simulink model "simulation_three_motors"  (R2022a)
settings: Solver=FixedStepAuto  StartTime=0.0  StopTime=inf  FixedStep=Ts  RelTol=1e-3
libraries: slDxl_lib_old x8
settings Model: Creator=jeihunl  LastModifiedBy=Matija
settings SolverCC: AlgebraicLoopSolver=TrustRegion
settings DataIOCC: ReturnWorkspaceOutputs=off
settings OptimizationCC: LifeSpan=inf
settings DebuggingCC: UnconnectedInputMsg=warning  UnconnectedOutputMsg=warning  UnconnectedLineMsg=warning  SFExecutionAtInitializationDiag=none  SFMachineParentedDataDiag=warning  ArithmeticOperatorsInVariantConditions=warning
settings HardwareCC: ProdBitPerSizeT=32  ProdBitPerPtrDiffT=32  ProdWordSize=32  ProdHWDeviceType=Specified
settings SFSimCC: SimUseLocalCustomCode=off  CustomCodeUndefinedFunction=UseInterfaceOnly
settings RTWCC: RTWUseLocalCustomCode=off
settings CodeAppCC: StateflowObjectComments=on

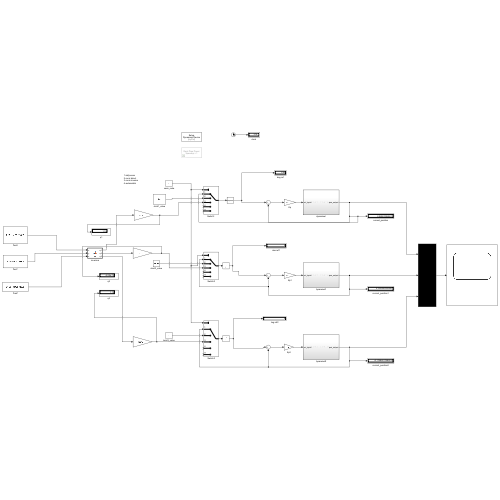
[thumbnail: Simulink's stored preview of the top-level diagram]
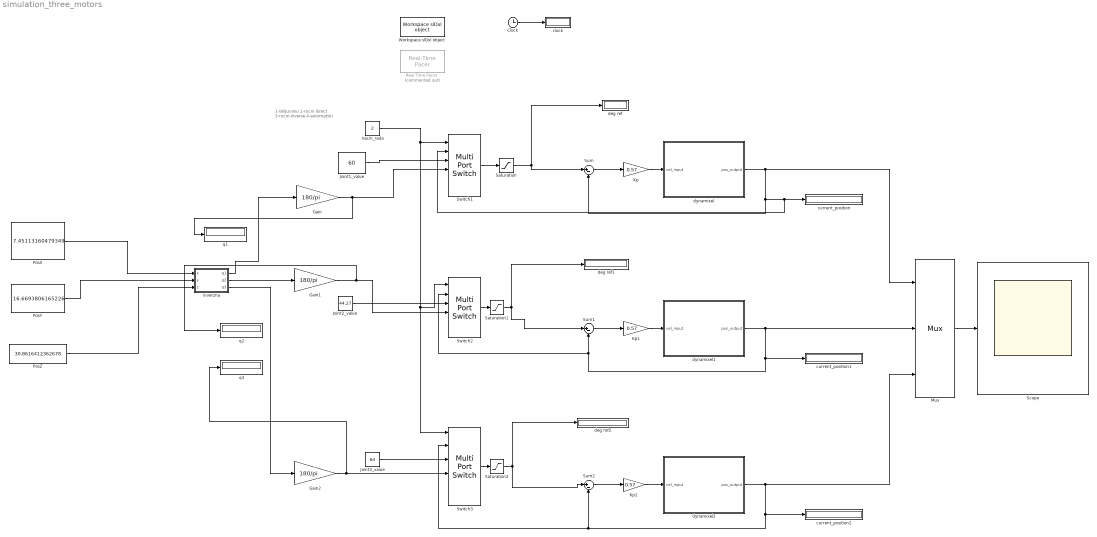
== system simulation_three_motors ==
  note: 1-iskljuceno
      | 2-rucni direct
      | 3-rucni-inverse
      | 4-automatski
  Clock : Clock
  Gain : Gain  Gain=180/pi
  Gain1 : Gain  Gain=180/pi
  Gain2 : Gain  Gain=180/pi
  Joint1_value : Constant  Value=60
  Joint2_value : Constant  Value=44.27
  Joint3_value : Constant  Value=64
  Kp : Gain  Gain=0.57
  Kp1 : Gain  Gain=0.57
  Kp2 : Gain  Gain=0.57
  Mux : Mux  Inputs=3
  PosX : Constant  Value=7.45113160479349  VectorParams1D=off  SampleTime=-1
  PosY : Constant  Value=16.6693806165226  VectorParams1D=off  SampleTime=-1
  PosZ : Constant  Value=30.8616412362678  VectorParams1D=off  SampleTime=-1
  Real-Time Pacer : slDxl_lib_old/Real-Time Pacer  Commented=on  simTimePerRealTime=1
  Saturation : Saturate  UpperLimit=180  LowerLimit=-180
  Saturation1 : Saturate  UpperLimit=100  LowerLimit=0
  Saturation2 : Saturate  UpperLimit=60  LowerLimit=0
  Scope : Scope
  Sum : Sum  Inputs=|+-
  Sum1 : Sum  Inputs=|+-
  Sum2 : Sum  Inputs=|+-
  "Switch1 " : MultiPortSwitch  Inputs=4  DataPortForDefault=Additional data port  SaturateOnIntegerOverflow=off  InputSameDT=off
  Switch2 : MultiPortSwitch  Inputs=4  DataPortForDefault=Additional data port  SaturateOnIntegerOverflow=off  InputSameDT=off
  Switch3 : MultiPortSwitch  Inputs=4  DataPortForDefault=Additional data port  SaturateOnIntegerOverflow=off  InputSameDT=off
  Workspace slDxl object : slDxl_lib_old/Workspace slDxl object  slDxlVarName=Existing Object Handle #1  workspaceVarName=myDxl
  clock : Display
  current_position : Display
      settings: Decimation=5
  current_position1 : Display
      settings: Decimation=5
  current_position2 : Display
      settings: Decimation=5
  deg ref : Display
  deg ref1 : Display
  deg ref2 : Display
  dynamixel : Subsystem
  dynamixel1 : Subsystem
  dynamixel2 : Subsystem
  inverzna : MATLAB Function  TreatAsAtomicUnit=on
  nacin_rada : Constant  Value=2
  q1 : Display
  q2 : Display
  q3 : Display
  wires:
  dynamixel/1(pos_output) -> Mux/1, Sum/2, "Switch1 "/2, current_position/1
  Sum/1 -> Kp/1
  Clock/1 -> clock/1
  Sum1/1 -> Kp1/1
  dynamixel1/1(pos_output) -> Mux/2, Switch2/2, Sum1/2, current_position1/1
  Kp1/1 -> dynamixel1/1(vel_input)
  Kp2/1 -> dynamixel2/1(vel_input)
  dynamixel2/1(pos_output) -> Mux/3, Switch3/2, Sum2/2, current_position2/1
  Sum2/1 -> Kp2/1
  Mux/1 -> Scope/1
  Kp/1 -> dynamixel/1(vel_input)
  "Switch1 "/1 -> Saturation/1
  Joint1_value/1 -> "Switch1 "/3
  nacin_rada/1 -> Switch3/1, Switch2/1, "Switch1 "/1
  Joint3_value/1 -> Switch3/3
  Switch3/1 -> Saturation2/1
  Joint2_value/1 -> Switch2/3
  Switch2/1 -> Saturation1/1
  PosX/1 -> inverzna/1(x)
  PosY/1 -> inverzna/2(y)
  PosZ/1 -> inverzna/3(z)
  inverzna/2(q2) -> Gain1/1
  inverzna/3(q3) -> Gain2/1
  inverzna/1(q1) -> Gain/1
  Gain/1 -> q1/1, "Switch1 "/4
  Gain1/1 -> q2/1, Switch2/4
  Gain2/1 -> q3/1, Switch3/4
  Saturation/1 -> Sum/1, deg ref/1
  Saturation1/1 -> Sum1/1, deg ref1/1
  Saturation2/1 -> Sum2/1, deg ref2/1

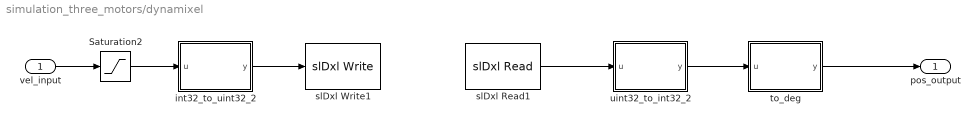
== system simulation_three_motors/dynamixel ==
  vel_input : Inport
  Saturation2 : Saturate  UpperLimit=256  LowerLimit=-256
  int32_to_uint32_2 : MATLAB Function  TreatAsAtomicUnit=on
  slDxl Read1 : slDxl_lib_old/slDxl Read  slDxlObject=Existing Object Handle #1  DXL_ID=1  DXL_ADDR=132  DXL_READ_SIZE=4  sampleT=Ts
  slDxl Write1 : slDxl_lib_old/slDxl Write  slDxlObject=Existing Object Handle #1  DXL_ID=1  DXL_ADDR=104  DXL_WRITE_SIZE=4  sampleT=Ts
  to_deg : MATLAB Function  TreatAsAtomicUnit=on
  uint32_to_int32_2 : MATLAB Function  TreatAsAtomicUnit=on
  pos_output : Outport  VectorParamsAs1DForOutWhenUnconnected=off
  wires:
  vel_input/1 -> Saturation2/1
  uint32_to_int32_2/1(y) -> to_deg/1(u)
  slDxl Read1/1 -> uint32_to_int32_2/1(u)
  Saturation2/1 -> int32_to_uint32_2/1(u)
  to_deg/1(y) -> pos_output/1
  int32_to_uint32_2/1(y) -> slDxl Write1/1

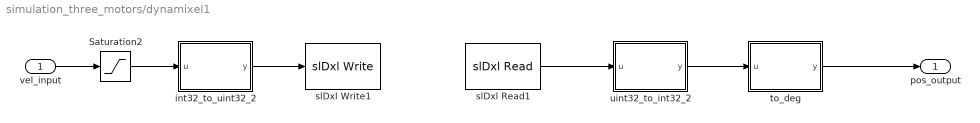
== system simulation_three_motors/dynamixel1 ==
  vel_input : Inport
  Saturation2 : Saturate  UpperLimit=256  LowerLimit=-256
  int32_to_uint32_2 : MATLAB Function  TreatAsAtomicUnit=on
  slDxl Read1 : slDxl_lib_old/slDxl Read  slDxlObject=Existing Object Handle #1  DXL_ID=2  DXL_ADDR=132  DXL_READ_SIZE=4  sampleT=Ts
  slDxl Write1 : slDxl_lib_old/slDxl Write  slDxlObject=Existing Object Handle #1  DXL_ID=2  DXL_ADDR=104  DXL_WRITE_SIZE=4  sampleT=Ts
  to_deg : MATLAB Function  TreatAsAtomicUnit=on
  uint32_to_int32_2 : MATLAB Function  TreatAsAtomicUnit=on
  pos_output : Outport  VectorParamsAs1DForOutWhenUnconnected=off
  wires:
  vel_input/1 -> Saturation2/1
  uint32_to_int32_2/1(y) -> to_deg/1(u)
  slDxl Read1/1 -> uint32_to_int32_2/1(u)
  Saturation2/1 -> int32_to_uint32_2/1(u)
  to_deg/1(y) -> pos_output/1
  int32_to_uint32_2/1(y) -> slDxl Write1/1

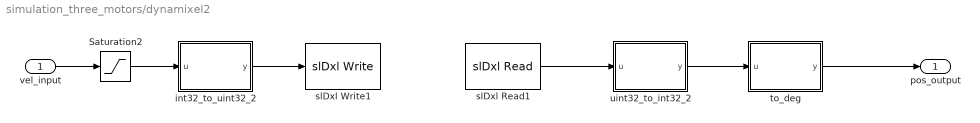
== system simulation_three_motors/dynamixel2 ==
  vel_input : Inport
  Saturation2 : Saturate  UpperLimit=256  LowerLimit=-256
  int32_to_uint32_2 : MATLAB Function  TreatAsAtomicUnit=on
  slDxl Read1 : slDxl_lib_old/slDxl Read  slDxlObject=Existing Object Handle #1  DXL_ID=3  DXL_ADDR=132  DXL_READ_SIZE=4  sampleT=Ts
  slDxl Write1 : slDxl_lib_old/slDxl Write  slDxlObject=Existing Object Handle #1  DXL_ID=3  DXL_ADDR=104  DXL_WRITE_SIZE=4  sampleT=Ts
  to_deg : MATLAB Function  TreatAsAtomicUnit=on
  uint32_to_int32_2 : MATLAB Function  TreatAsAtomicUnit=on
  pos_output : Outport  VectorParamsAs1DForOutWhenUnconnected=off
  wires:
  vel_input/1 -> Saturation2/1
  uint32_to_int32_2/1(y) -> to_deg/1(u)
  slDxl Read1/1 -> uint32_to_int32_2/1(u)
  Saturation2/1 -> int32_to_uint32_2/1(u)
  to_deg/1(y) -> pos_output/1
  int32_to_uint32_2/1(y) -> slDxl Write1/1

== matlab function simulation_three_motors/dynamixel/uint32_to_int32_2 ==
  data: u input; y output
function y = fcn(u)
    temp = typecast(uint32(u), 'int32');
    y = double(temp(1));
end

== matlab function simulation_three_motors/dynamixel1/int32_to_uint32_2 ==
  data: u input; y output
function y = fcn(u)
    temp = typecast(int32(u), 'uint32');
    y = temp(1);
end

== matlab function simulation_three_motors/dynamixel/to_deg ==
  data: u input; y output
function y = fcn(u)
    y = (u / 4095.0) * 360.0;
end

== matlab function simulation_three_motors/dynamixel/int32_to_uint32_2 ==
  data: u input; y output
function y = fcn(u)
    temp = typecast(int32(u), 'uint32');
    y = temp(1);
end

== matlab function simulation_three_motors/dynamixel1/to_deg ==
  data: u input; y output
function y = fcn(u)
    y = (u / 4095.0) * 360.0;
end

== matlab function simulation_three_motors/dynamixel1/uint32_to_int32_2 ==
  data: u input; y output
function y = fcn(u)
    temp = typecast(uint32(u), 'int32');
    y = double(temp(1));
end

== matlab function simulation_three_motors/dynamixel2/int32_to_uint32_2 ==
  data: u input; y output
function y = fcn(u)
    temp = typecast(int32(u), 'uint32');
    y = temp(1);
end

== matlab function simulation_three_motors/dynamixel2/to_deg ==
  data: u input; y output
function y = fcn(u)
    y = (u / 4095.0) * 360.0;
end

== matlab function simulation_three_motors/dynamixel2/uint32_to_int32_2 ==
  data: u input; y output
function y = fcn(u)
    temp = typecast(uint32(u), 'int32');
    y = double(temp(1));
end

== matlab function simulation_three_motors/inverzna ==
  data: x input; q1 output; y input; z input; q2 output; q3 output
function [q1,q2,q3] = fcn(x,y,z)
a1 = 8.2-1.5;
a2 = 16;        %%cm
a3 = 20;

q1 = atan2(y,x);
q3 = acos((x^2+y^2+(z-a1)^2-a2^2-a3^2)/(2*a2*a3));
q2 = pi/2 -atan2(z-a1, sqrt(x^2+y^2)) - atan2(sin(q3)*a3, a2+cos(q3)*a3);
